simulink model "ex2"  (R2025a)
settings: Solver=VariableStepAuto  StartTime=0.0  StopTime=T0  MaxStep=dt  RelTol=tol
InitFcn:
  | init
values from neighbouring files (symbols this model uses):
  I = [Ix  0  0 ... (first row only)    [init.m]
  K_phi = status(1)    [init.m]
  K_psi = status(1)    [init.m]
  K_theta = status(1)    [init.m]
  omegaBI_IC = [0;-omega_OI;0]    [init.m]
  q_IC = [0; 0; 0; 1]    [init.m]
  T1_phi = status(2)    [init.m]
  T1_psi = status(2)    [init.m]
  T1_theta = status(2)    [init.m]
  T2_phi = status(3)    [init.m]
  T2_psi = status(3)    [init.m]
  T2_theta = status(3)    [init.m]
settings Model: Creator=comumar20700  LastModifiedBy=modeand16864

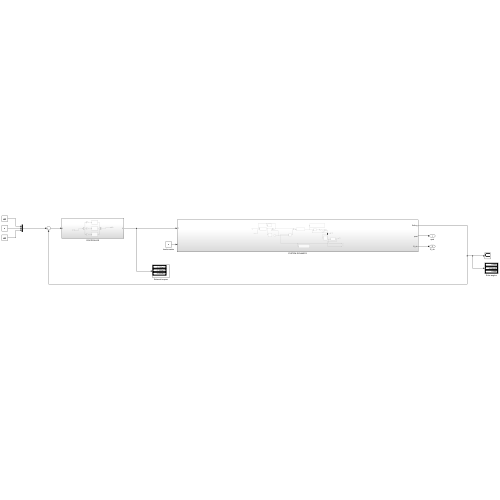
[thumbnail: Simulink's stored preview of the top-level diagram]
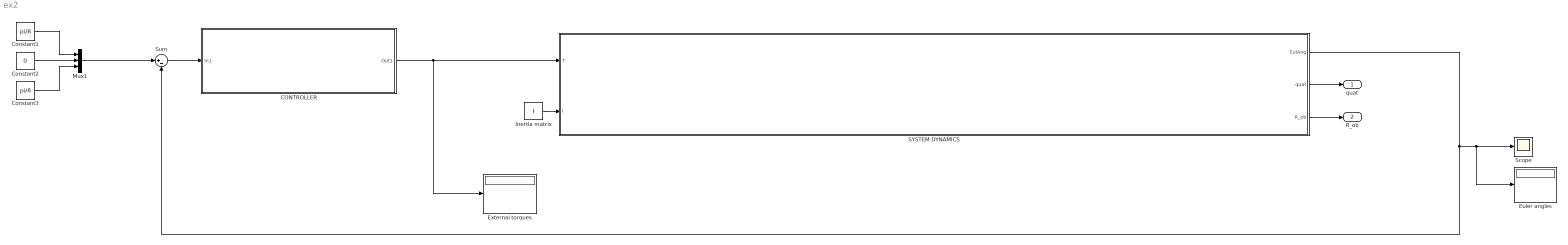
== system ex2 ==
  CONTROLLER : Subsystem
  Constant1 : Constant  Value=pi/8
  Constant2 : Constant  Value=0
  Constant3 : Constant  Value=pi/8
  Euler angles : Display
  External torques : Display
  Inertia matrix : Constant  Value=I
  Mux1 : Mux  Inputs=3
  SYSTEM DYNAMICS : Subsystem
  Scope : Scope
      settings: ActiveDisplayYMinimum=-0.82948068859602908  ActiveDisplayYMaximum=1.6383540749786294  DataLoggingVariableName=ScopeData2
  Sum : Sum  Inputs=|+-
  quat : Outport
  R_ob : Outport  Port=2
  wires:
  Mux1/1 -> Sum/1
  Constant3/1 -> Mux1/3
  Constant2/1 -> Mux1/2
  Constant1/1 -> Mux1/1
  CONTROLLER/1(Out1) -> External torques/1, SYSTEM DYNAMICS/1(T)
  Sum/1 -> CONTROLLER/1(In1)
  SYSTEM DYNAMICS/1(EulAng) -> Sum/2, Euler angles/1, Scope/1
  Inertia matrix/1 -> SYSTEM DYNAMICS/2(I)
  SYSTEM DYNAMICS/2(quat) -> quat/1
  SYSTEM DYNAMICS/3(R_ob) -> R_ob/1

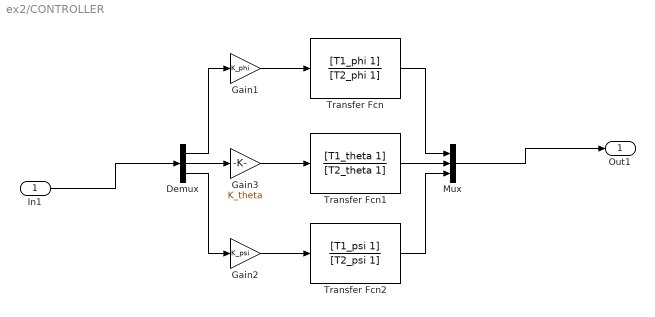
== system ex2/CONTROLLER ==
  In1 : Inport
  Demux : Demux  Outputs=3
  Gain1 : Gain  Gain=K_phi
  Gain2 : Gain  Gain=K_psi
  Gain3 : Gain  Gain=K_theta
  Mux : Mux  Inputs=3
  Transfer Fcn : TransferFcn  Numerator=[T1_phi 1]  Denominator=[T2_phi 1]
  Transfer Fcn1 : TransferFcn  Numerator=[T1_theta 1]  Denominator=[T2_theta 1]
  Transfer Fcn2 : TransferFcn  Numerator=[T1_psi 1]  Denominator=[T2_psi 1]
  Out1 : Outport
  wires:
  Transfer Fcn1/1 -> Mux/2
  Gain1/1 -> Transfer Fcn/1
  Transfer Fcn2/1 -> Mux/3
  Gain2/1 -> Transfer Fcn2/1
  Transfer Fcn/1 -> Mux/1
  Gain3/1 -> Transfer Fcn1/1
  Demux/1 -> Gain1/1
  Demux/3 -> Gain2/1
  Demux/2 -> Gain3/1
  Mux/1 -> Out1/1
  In1/1 -> Demux/1

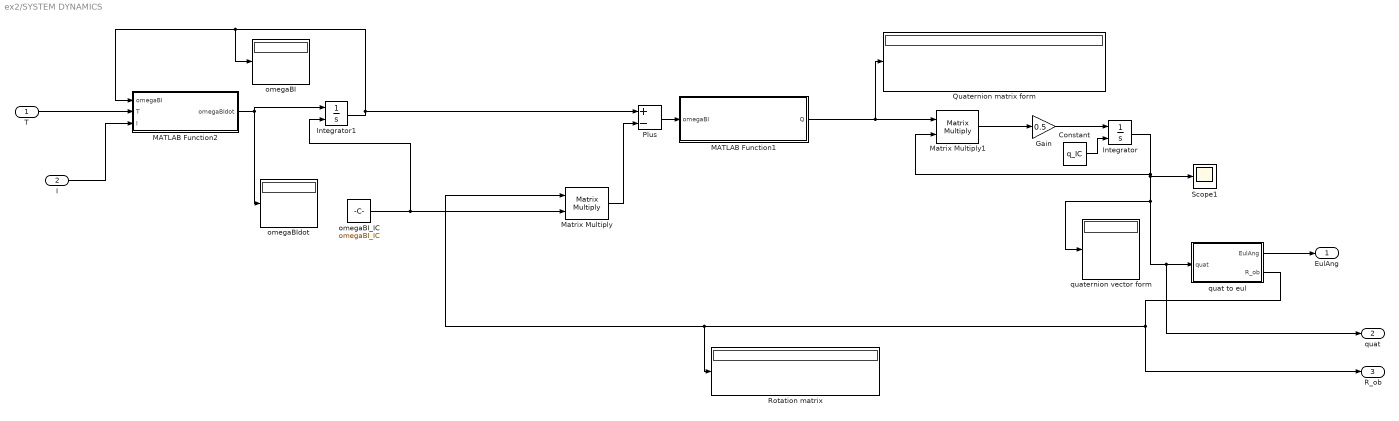
== system ex2/SYSTEM DYNAMICS ==
  T : Inport
  I : Inport  Port=2
  Constant : Constant  Value=q_IC
  Gain : Gain  Gain=0.5
  Integrator : Integrator  InitialConditionSource=external  InitialCondition=q_IC
  Integrator1 : Integrator  InitialConditionSource=external  InitialCondition=omegaBI_IC
  MATLAB Function1 : MATLAB Function  TreatAsAtomicUnit=on
  MATLAB Function2 : MATLAB Function  TreatAsAtomicUnit=on
  Matrix Multiply : Product  Multiplication=Matrix(*)
  Matrix Multiply1 : Product  Multiplication=Matrix(*)
  Plus : Sum  Inputs=+-
  Quaternion matrix form : Display
  Rotation matrix : Display
  Scope1 : Scope
      settings: ActiveDisplayYMinimum=-0.668977773659647  ActiveDisplayYMaximum=1.7853288413912287  DataLoggingVariableName=ScopeData3
  omegaBI : Display
  omegaBI_IC : Constant  Value=omegaBI_IC
  omegaBIdot : Display
  quat to eul : Subsystem
  quaternion vector form : Display
  EulAng : Outport
  quat : Outport  Port=2
  R_ob : Outport  Port=3
  wires:
  Matrix Multiply1/1 -> Gain/1
  Matrix Multiply/1 -> Plus/2
  MATLAB Function1/1(Q) -> Matrix Multiply1/1, Quaternion matrix form/1
  MATLAB Function2/1(omegaBIdot) -> Integrator1/1, omegaBIdot/1
  Gain/1 -> Integrator/1
  quat to eul/2(R_ob) -> R_ob/1, Matrix Multiply/1, Rotation matrix/1
  I/1 -> MATLAB Function2/3(I)
  Plus/1 -> MATLAB Function1/1(omegaBI)
  omegaBI_IC/1 -> Integrator1/2, Matrix Multiply/2
  Constant/1 -> Integrator/2
  Integrator1/1 -> Plus/1, MATLAB Function2/1(omegaBI), omegaBI/1
  Integrator/1 -> quaternion vector form/1, quat/1, quat to eul/1(quat), Scope1/1, Matrix Multiply1/2
  quat to eul/1(EulAng) -> EulAng/1
  T/1 -> MATLAB Function2/2(T)

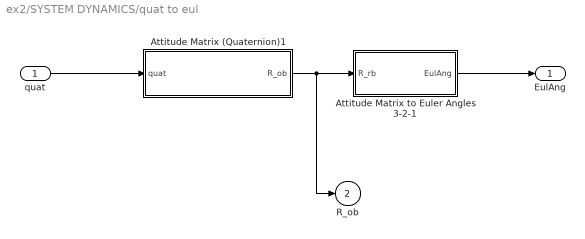
== system ex2/SYSTEM DYNAMICS/quat to eul ==
  quat : Inport
  Attitude Matrix (Quaternion)1 : Subsystem
  Attitude Matrix to Euler Angles 3-2-1 : Subsystem
  EulAng : Outport  VectorParamsAs1DForOutWhenUnconnected=off
  R_ob : Outport  Port=2
  wires:
  Attitude Matrix to Euler Angles 3-2-1/1(EulAng) -> EulAng/1
  Attitude Matrix (Quaternion)1/1(R_ob) -> Attitude Matrix to Euler Angles 3-2-1/1(R_rb), R_ob/1
  quat/1 -> Attitude Matrix (Quaternion)1/1(quat)

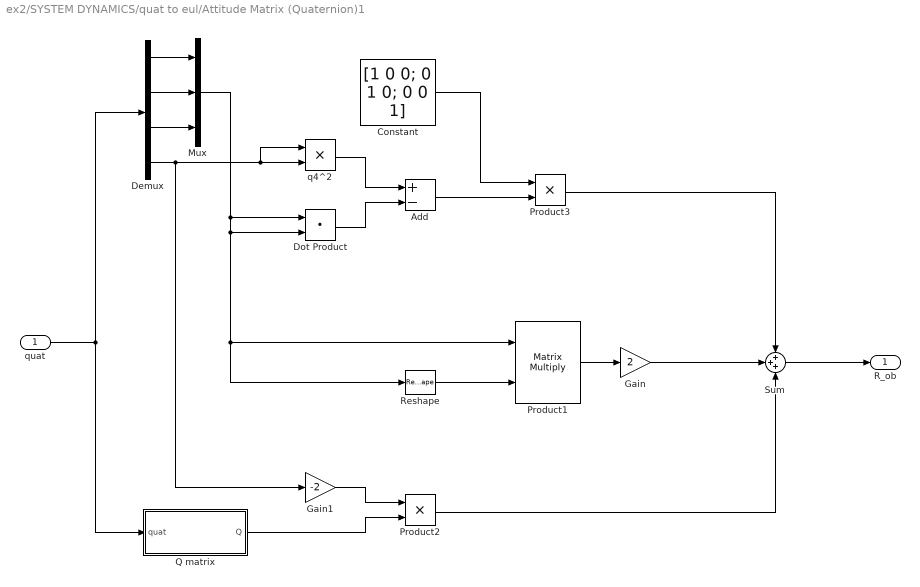
== system ex2/SYSTEM DYNAMICS/quat to eul/Attitude Matrix (Quaternion)1 ==
  quat : Inport
  Add : Sum  Inputs=+-
  Constant : Constant  Value=[1 0 0; 0 1 0; 0 0 1]
  Demux : Demux
  Dot Product : DotProduct  OutDataTypeStr=Inherit: Inherit via internal rule
  Gain : Gain  Gain=2
  Gain1 : Gain  Gain=-2
  Mux : Mux  Inputs=3
  Product1 : Product  Multiplication=Matrix(*)  RndMeth=Zero
  Product2 : Product  RndMeth=Zero
  Product3 : Product  RndMeth=Zero
  Q matrix : Subsystem
  Reshape : Reshape  OutputDimensionality=Row vector (2-D)
  Sum : Sum  Inputs=+++
  q4^2 : Product  RndMeth=Zero
  R_ob : Outport  VectorParamsAs1DForOutWhenUnconnected=off
  wires:
  quat/1 -> Demux/1, Q matrix/1(quat)
  Demux/4 -> q4^2/2, q4^2/1, Gain1/1
  Reshape/1 -> Product1/2
  Product1/1 -> Gain/1
  Gain/1 -> Sum/2
  q4^2/1 -> Add/1
  Dot Product/1 -> Add/2
  Product2/1 -> Sum/3
  Add/1 -> Product3/2
  Sum/1 -> R_ob/1
  Constant/1 -> Product3/1
  Product3/1 -> Sum/1
  Demux/1 -> Mux/1
  Demux/2 -> Mux/2
  Demux/3 -> Mux/3
  Mux/1 -> Dot Product/1, Reshape/1, Product1/1, Dot Product/2
  Gain1/1 -> Product2/1
  Q matrix/1(Q) -> Product2/2

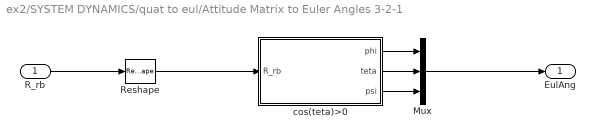
== system ex2/SYSTEM DYNAMICS/quat to eul/Attitude Matrix to Euler Angles 3-2-1 ==
  R_rb : Inport
  Mux : Mux  Inputs=3
  Reshape : Reshape  OutputDimensionality=Column vector (2-D)
  cos(teta)>0 : Subsystem
  EulAng : Outport  VectorParamsAs1DForOutWhenUnconnected=off
  wires:
  cos(teta)>0/2(teta) -> Mux/2
  cos(teta)>0/1(phi) -> Mux/1
  cos(teta)>0/3(psi) -> Mux/3
  Mux/1 -> EulAng/1
  Reshape/1 -> cos(teta)>0/1(R_rb)
  R_rb/1 -> Reshape/1

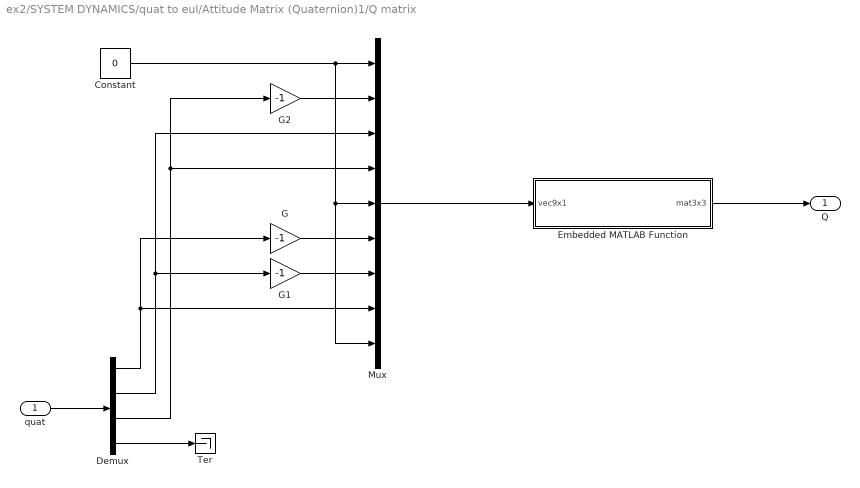
== system ex2/SYSTEM DYNAMICS/quat to eul/Attitude Matrix (Quaternion)1/Q matrix ==
  quat : Inport
  Constant : Constant  Value=0
  Demux : Demux
  Embedded MATLAB Function : MATLAB Function  TreatAsAtomicUnit=on
  G : Gain  Gain=-1
  G1 : Gain  Gain=-1
  G2 : Gain  Gain=-1
  Mux : Mux  Inputs=9
  Ter : Terminator
  Q : Outport  VectorParamsAs1DForOutWhenUnconnected=off
  wires:
  Demux/4 -> Ter/1
  quat/1 -> Demux/1
  Constant/1 -> Mux/9, Mux/5, Mux/1
  Demux/1 -> G/1, Mux/8
  G1/1 -> Mux/7
  Demux/2 -> G1/1, Mux/3
  G/1 -> Mux/6
  G2/1 -> Mux/2
  Demux/3 -> G2/1, Mux/4
  Embedded MATLAB Function/1(mat3x3) -> Q/1
  Mux/1 -> Embedded MATLAB Function/1(vec9x1)

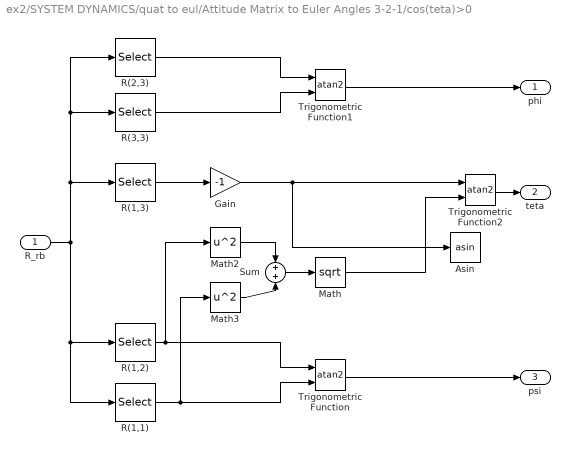
== system ex2/SYSTEM DYNAMICS/quat to eul/Attitude Matrix to Euler Angles 3-2-1/cos(teta)>0 ==
  R_rb : Inport
  Asin : Trigonometry  Operator=asin
  Gain : Gain  Gain=-1
  Math : Math  Operator=sqrt  SignedPower=on
  Math2 : Math  Operator=square  SignedPower=on
  Math3 : Math  Operator=square  SignedPower=on
  R(1,1) : Selector  InputPortWidth=9  IndexOptions=Index vector (dialog)  Indices=[1]  OutputSizes=1
  R(1,2) : Selector  InputPortWidth=9  IndexOptions=Index vector (dialog)  Indices=[4]  OutputSizes=1
  R(1,3) : Selector  InputPortWidth=9  IndexOptions=Index vector (dialog)  Indices=[7]  OutputSizes=1
  R(2,3) : Selector  InputPortWidth=9  IndexOptions=Index vector (dialog)  Indices=[8]  OutputSizes=1
  R(3,3) : Selector  InputPortWidth=9  IndexOptions=Index vector (dialog)  Indices=[9]  OutputSizes=1
  Sum : Sum
  Trigonometric Function : Trigonometry  Operator=atan2
  Trigonometric Function1 : Trigonometry  Operator=atan2
  Trigonometric Function2 : Trigonometry  Operator=atan2
  phi : Outport  VectorParamsAs1DForOutWhenUnconnected=off
  teta : Outport  Port=2  VectorParamsAs1DForOutWhenUnconnected=off
  psi : Outport  Port=3  VectorParamsAs1DForOutWhenUnconnected=off
  wires:
  R_rb/1 -> R(1,1)/1, R(1,2)/1, R(1,3)/1, R(3,3)/1, R(2,3)/1
  R(1,2)/1 -> Trigonometric Function/1, Math2/1
  R(1,1)/1 -> Trigonometric Function/2, Math3/1
  R(2,3)/1 -> Trigonometric Function1/1
  R(3,3)/1 -> Trigonometric Function1/2
  R(1,3)/1 -> Gain/1
  Gain/1 -> Asin/1, Trigonometric Function2/1
  Math2/1 -> Sum/1
  Math3/1 -> Sum/2
  Sum/1 -> Math/1
  Math/1 -> Trigonometric Function2/2
  Trigonometric Function1/1 -> phi/1
  Trigonometric Function2/1 -> teta/1
  Trigonometric Function/1 -> psi/1

== matlab function ex2/SYSTEM DYNAMICS/MATLAB Function1 ==
  data: omegaBI input; Q output
function Q = fcn(omegaBI)

omegaBIx = omegaBI(1);
omegaBIy = omegaBI(2);
omegaBIz = omegaBI(3);

Q=[        0  omegaBIz -omegaBIy  omegaBIx;
   -omegaBIz         0  omegaBIx  omegaBIy;
    omegaBIy -omegaBIx         0  omegaBIz;
   -omegaBIx -omegaBIy -omegaBIz         0];

== matlab function ex2/SYSTEM DYNAMICS/MATLAB Function2 ==
  data: omegaBI input; T input; I input; omegaBIdot output
function omegaBIdot = fcn(omegaBI, T, I)

omegaBIdot = I'*(T-cross(omegaBI, I*omegaBI));

== matlab function ex2/SYSTEM DYNAMICS/quat to eul/Attitude Matrix (Quaternion)1/Q matrix/Embedded MATLAB Function ==
  data: vec9x1 input; mat3x3 output
function mat3x3 = vec2mat(vec9x1)
%#eml

s = size(vec9x1);

if s(1)>s(2)
    vec = vec9x1';
else
    vec = vec9x1;
end

mat3x3 = [vec(1:3); vec(4:6); vec(7:9)];
